simulink model "Cockpit"  (R2012b)
settings: Solver=ode45  StartTime=0.0  StopTime=10.0  RelTol=1e-3
undefined symbols (not defined in the file or in its folder): sigbuilder_block
libraries: vrlib x1
settings Model: Creator=David  LastModifiedBy=David

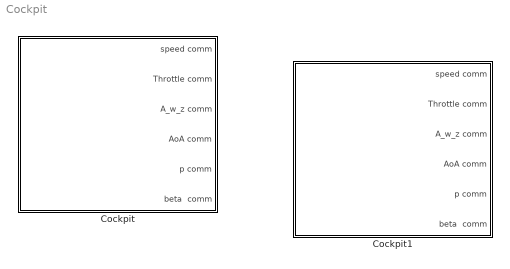
== system Cockpit ==
  Cockpit : Subsystem
      mask Display:
      | image(imread('Cockpit2.jpg'))
      | 
      | 
      | port_label('output', 1, 'Speed comm')
      | port_label('output', 2, 'Throttle comm')
      | port_label('output', 3, 'A_w_z comm')
      | port_label('output', 4, 'AoA comm')
      | port_label('output', 5, 'p comm')
      | port_label('output', 6, 'beta comm')
  Cockpit1 : Subsystem
      mask Display:
      | image(imread('Cockpit2.jpg'))
      | 
      | 
      | port_label('output', 1, 'Speed comm')
      | port_label('output', 2, 'Throttle comm')
      | port_label('output', 3, 'A_w_z comm')
      | port_label('output', 4, 'AoA comm')
      | port_label('output', 5, 'p comm')
      | port_label('output', 6, 'beta comm')

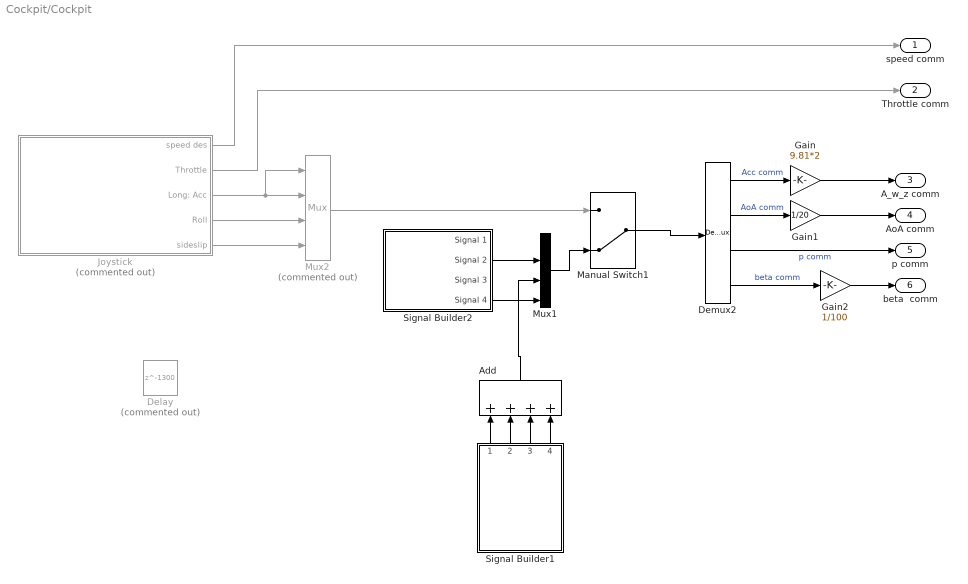
== system Cockpit/Cockpit ==
  Add : Sum  Inputs=++++
  Delay : Delay  Commented=on  DelayLength=1300
  Demux2 : Demux
  Gain : Gain  Gain=9.81*2
  Gain1 : Gain  Gain=1/20
  Gain2 : Gain  Gain=1/100
  Joystick : Subsystem  Commented=on
  Manual Switch1 : ManualSwitch  CurrentSetting=0
  Mux1 : Mux
  Mux2 : Mux  Commented=on
  Signal Builder1 : Subsystem  Tag=STV Subsys  LoadFcn=sigbuilder_block('load');  StartFcn=sigbuilder_block('start');  StopFcn=sigbuilder_block('stop');  ClipboardFcn=sigbuilder_block('clipboard');  mask(Sigbuilder block){}
      mask help: Simulink:masks:SigbuilderBlock_MD
      mask init:
      | if ~strcmp(get_param(bdroot(gcbh),'SimulationStatus'),'stopped') tuvar = sigbuilder_block('maskInit'); end
      settings: CopyFcn=sigbuilder_block('copy');  DeleteFcn=sigbuilder_block('delete');  ModelCloseFcn=sigbuilder_block('modelClose');  PreSaveFcn=sigbuilder_block('preSave');  PauseFcn=sigbuilder_block('pause');  ContinueFcn=sigbuilder_block('continue');  NameChangeFcn=sigbuilder_block('namechange');  OpenFcn=sigbuilder_block('open',[0 30 1024.5 489 ]);  CloseFcn=sigbuilder_block('close');
      mask Display: plot(0, 0, 100, 100,[2, 2, 32, 32, 2], [68, 8, 8, 68, 68],[32, 2], [38, 38], [32, 19, 2],[53, 60, 44], [32, 17, 17, 2],[16, 16, 31, 31]);txt = getActiveGroup(gcbh);text(2, 100, txt,'verticalAlignment', 'top');
  Signal Builder2 : Subsystem  Tag=STV Subsys  LoadFcn=sigbuilder_block('load');  StartFcn=sigbuilder_block('start');  StopFcn=sigbuilder_block('stop');  ClipboardFcn=sigbuilder_block('clipboard');  mask(Sigbuilder block){}
      mask help: Simulink:masks:SigbuilderBlock_MD
      mask init:
      | if ~strcmp(get_param(bdroot(gcbh),'SimulationStatus'),'stopped') tuvar = sigbuilder_block('maskInit'); end
      settings: CopyFcn=sigbuilder_block('copy');  DeleteFcn=sigbuilder_block('delete');  ModelCloseFcn=sigbuilder_block('modelClose');  PreSaveFcn=sigbuilder_block('preSave');  PauseFcn=sigbuilder_block('pause');  ContinueFcn=sigbuilder_block('continue');  NameChangeFcn=sigbuilder_block('namechange');  OpenFcn=sigbuilder_block('open',[6 28.5 1012.5 484.5 ]);  CloseFcn=sigbuilder_block('close');
      mask Display: plot(0, 0, 100, 100,[2, 2, 32, 32, 2], [68, 8, 8, 68, 68],[32, 2], [38, 38], [32, 19, 2],[53, 60, 44], [32, 17, 17, 2],[16, 16, 31, 31]);txt = getActiveGroup(gcbh);text(2, 100, txt,'verticalAlignment', 'top');
  speed comm : Outport
  Throttle comm : Outport  Port=2
  A_w_z comm : Outport  Port=3
  AoA comm : Outport  Port=4
  p comm : Outport  Port=5
  beta  comm : Outport  Port=6
  wires:
  Demux2/2 -> Gain1/1  "AoA comm"
  Gain/1 -> A_w_z comm/1
  Mux1/1 -> Manual Switch1/2
  Manual Switch1/1 -> Demux2/1
  Demux2/1 -> Gain/1  "Acc comm"
  Demux2/3 -> p comm/1  "p comm"
  Demux2/4 -> Gain2/1  "beta comm"
  Joystick/5(sideslip) -> Mux2/4
  Joystick/4(Roll) -> Mux2/3
  Joystick/2(Throttle) -> Throttle comm/1
  Mux2/1 -> Manual Switch1/1
  Joystick/3(Long: Acc) -> Mux2/1, Mux2/2
  Gain1/1 -> AoA comm/1
  Signal Builder1/1(Signal 1) -> Add/1
  Signal Builder1/2(Signal 5) -> Add/2
  Signal Builder1/4(Signal 7) -> Add/4
  Signal Builder1/3(Signal 6) -> Add/3
  Gain2/1 -> beta  comm/1
  Signal Builder2/2(Signal 2) -> Mux1/2
  Signal Builder2/4(Signal 4) -> Mux1/4
  Joystick/1(speed des) -> speed comm/1
  Add/1 -> Mux1/3

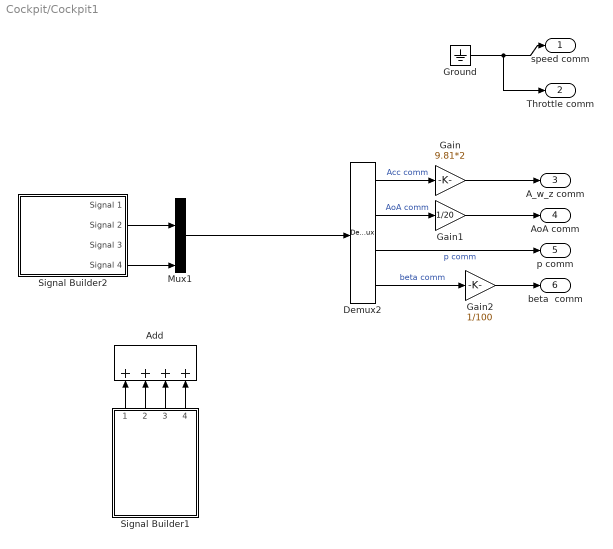
== system Cockpit/Cockpit1 ==
  Add : Sum  Inputs=++++
  Demux2 : Demux
  Gain : Gain  Gain=9.81*2
  Gain1 : Gain  Gain=1/20
  Gain2 : Gain  Gain=1/100
  Ground : Ground
  Mux1 : Mux
  Signal Builder1 : Subsystem  Tag=STV Subsys  LoadFcn=sigbuilder_block('load');  StartFcn=sigbuilder_block('start');  StopFcn=sigbuilder_block('stop');  ClipboardFcn=sigbuilder_block('clipboard');  mask(Sigbuilder block){}
      mask help: Simulink:masks:SigbuilderBlock_MD
      mask init:
      | if ~strcmp(get_param(bdroot(gcbh),'SimulationStatus'),'stopped') tuvar = sigbuilder_block('maskInit'); end
      settings: CopyFcn=sigbuilder_block('copy');  DeleteFcn=sigbuilder_block('delete');  ModelCloseFcn=sigbuilder_block('modelClose');  PreSaveFcn=sigbuilder_block('preSave');  PauseFcn=sigbuilder_block('pause');  ContinueFcn=sigbuilder_block('continue');  NameChangeFcn=sigbuilder_block('namechange');  OpenFcn=sigbuilder_block('open',[0 30 1024.5 489 ]);  CloseFcn=sigbuilder_block('close');
      mask Display: plot(0, 0, 100, 100,[2, 2, 32, 32, 2], [68, 8, 8, 68, 68],[32, 2], [38, 38], [32, 19, 2],[53, 60, 44], [32, 17, 17, 2],[16, 16, 31, 31]);txt = getActiveGroup(gcbh);text(2, 100, txt,'verticalAlignment', 'top');
  Signal Builder2 : Subsystem  Tag=STV Subsys  LoadFcn=sigbuilder_block('load');  StartFcn=sigbuilder_block('start');  StopFcn=sigbuilder_block('stop');  ClipboardFcn=sigbuilder_block('clipboard');  mask(Sigbuilder block){}
      mask help: Simulink:masks:SigbuilderBlock_MD
      mask init:
      | if ~strcmp(get_param(bdroot(gcbh),'SimulationStatus'),'stopped') tuvar = sigbuilder_block('maskInit'); end
      settings: CopyFcn=sigbuilder_block('copy');  DeleteFcn=sigbuilder_block('delete');  ModelCloseFcn=sigbuilder_block('modelClose');  PreSaveFcn=sigbuilder_block('preSave');  PauseFcn=sigbuilder_block('pause');  ContinueFcn=sigbuilder_block('continue');  NameChangeFcn=sigbuilder_block('namechange');  OpenFcn=sigbuilder_block('open',[6 28.5 1012.5 484.5 ]);  CloseFcn=sigbuilder_block('close');
      mask Display: plot(0, 0, 100, 100,[2, 2, 32, 32, 2], [68, 8, 8, 68, 68],[32, 2], [38, 38], [32, 19, 2],[53, 60, 44], [32, 17, 17, 2],[16, 16, 31, 31]);txt = getActiveGroup(gcbh);text(2, 100, txt,'verticalAlignment', 'top');
  speed comm : Outport
  Throttle comm : Outport  Port=2
  A_w_z comm : Outport  Port=3
  AoA comm : Outport  Port=4
  p comm : Outport  Port=5
  beta  comm : Outport  Port=6
  wires:
  Demux2/2 -> Gain1/1  "AoA comm"
  Gain/1 -> A_w_z comm/1
  Mux1/1 -> Demux2/1
  Demux2/1 -> Gain/1  "Acc comm"
  Demux2/3 -> p comm/1  "p comm"
  Demux2/4 -> Gain2/1  "beta comm"
  Gain1/1 -> AoA comm/1
  Signal Builder1/1(Signal 1) -> Add/1
  Signal Builder1/2(Signal 5) -> Add/2
  Signal Builder1/4(Signal 7) -> Add/4
  Signal Builder1/3(Signal 6) -> Add/3
  Gain2/1 -> beta  comm/1
  Signal Builder2/2(Signal 2) -> Mux1/2
  Signal Builder2/4(Signal 4) -> Mux1/4
  ? -> Mux1/3
  Ground/1 -> Throttle comm/1, speed comm/1

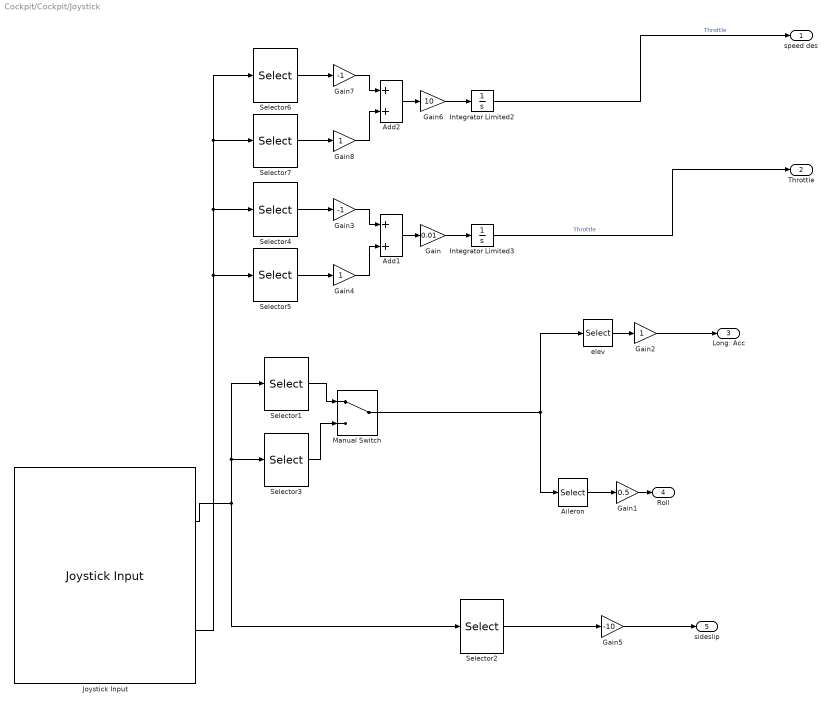
== system Cockpit/Cockpit/Joystick ==
  Add1 : Sum
  Add2 : Sum
  Aileron : Selector  InputPortWidth=2  IndexOptions=Index vector (dialog)  Indices=1  OutputSizes=1
  Gain : Gain  Gain=0.01  OutDataTypeStr=double
  Gain1 : Gain  Gain=0.5
  Gain2 : Gain
  Gain3 : Gain  Gain=-1
  Gain4 : Gain
  Gain5 : Gain  Gain=-10
  Gain6 : Gain  Gain=10  OutDataTypeStr=double
  Gain7 : Gain  Gain=-1
  Gain8 : Gain
  Integrator Limited2 : Integrator  LimitOutput=on  UpperSaturationLimit=400  LowerSaturationLimit=-400
  Integrator Limited3 : Integrator  LimitOutput=on  UpperSaturationLimit=1  LowerSaturationLimit=-1
  Joystick Input : vrlib/Joystick Input  joyid=1  adjustports=on  forcefeed=off
  Manual Switch : ManualSwitch
  Selector1 : Selector  InputPortWidth=5  IndexOptions=Index vector (dialog)  Indices=1:2  OutputSizes=1
  Selector2 : Selector  InputPortWidth=5  IndexOptions=Index vector (dialog)  Indices=3  OutputSizes=1
  Selector3 : Selector  InputPortWidth=5  IndexOptions=Index vector (dialog)  Indices=4:5  OutputSizes=1
  Selector4 : Selector  InputPortWidth=10  IndexOptions=Index vector (dialog)  Indices=1  OutputSizes=1
  Selector5 : Selector  InputPortWidth=10  IndexOptions=Index vector (dialog)  Indices=4  OutputSizes=1
  Selector6 : Selector  InputPortWidth=10  IndexOptions=Index vector (dialog)  Indices=1  OutputSizes=1
  Selector7 : Selector  InputPortWidth=10  IndexOptions=Index vector (dialog)  Indices=4  OutputSizes=1
  elev : Selector  InputPortWidth=2  IndexOptions=Index vector (dialog)  Indices=2  OutputSizes=1
  speed des : Outport
  Throttle : Outport  Port=2
  Long: Acc : Outport  Port=3
  Roll : Outport  Port=4
  sideslip : Outport  Port=5
  wires:
  Integrator Limited3/1 -> Throttle/1  "Throttle"
  Aileron/1 -> Gain1/1
  Manual Switch/1 -> Aileron/1, elev/1
  Joystick Input/1 -> Selector2/1, Selector3/1, Selector1/1
  Selector1/1 -> Manual Switch/1
  Selector3/1 -> Manual Switch/2
  Selector4/1 -> Gain3/1
  Selector5/1 -> Gain4/1
  Gain3/1 -> Add1/1
  Gain4/1 -> Add1/2
  Add1/1 -> Gain/1
  Gain/1 -> Integrator Limited3/1
  elev/1 -> Gain2/1
  Gain1/1 -> Roll/1
  Selector2/1 -> Gain5/1
  Gain2/1 -> Long: Acc/1
  Gain5/1 -> sideslip/1
  Integrator Limited2/1 -> speed des/1  "Throttle"
  Joystick Input/2 -> Selector5/1, Selector7/1, Selector6/1, Selector4/1
  Selector6/1 -> Gain7/1
  Selector7/1 -> Gain8/1
  Gain7/1 -> Add2/1
  Gain8/1 -> Add2/2
  Add2/1 -> Gain6/1
  Gain6/1 -> Integrator Limited2/1

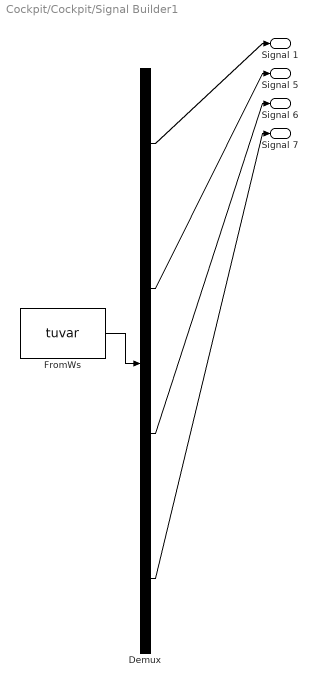
== system Cockpit/Cockpit/Signal Builder1 ==
  Demux : Demux  Tag=STV Demux
  FromWs : FromWorkspace  Tag=STV FromWs  VariableName=tuvar  SampleTime=0
      SigBuilderData=|
      | common.afterFinalStr = 'Extrapolate'
      | common.sampleTime = 0
      | dataSet.timeRange = [0 30]
      | dataSet.name = 'Group 1'
      | sbobj.Groups.Name = 'Group 1'
      | sbobj.Groups.Signals(1).Name = 'Signal 1'
      | sbobj.Groups.Signals(1).XData = [0 0.5 0.5 2.5 2.5 30]
      | sbobj.Groups.Signals(1).YData = [0 0 -1 -1 0 0]
      | sbobj.Groups.Signals(2).Name = 'Signal 5'
      | sbobj.Groups.Signals(2).XData = [0 4 4 6 6 30]
      | sbobj.Groups.Signals(2).YData = [0 0 1 1 0 0]
      | sbobj.Groups.Signals(3).Name = 'Signal 6'
      | sbobj.Groups.Signals(3).XData = [0 8 8 10 10 30]
      | sbobj.Groups.Signals(3).YData = [0 0 -0.5 -0.5 0 0]
      | sbobj.Groups.Signals(4).Name = 'Signal 7'
      | sbobj.Groups.Signals(4).XData = [0 12 12 14 14 30]
      | sbobj.Groups.Signals(4).YData = [0 0 0.5 0.5 0 0]
      | sbobj.Groups.TimeRange = [0 30]
  Signal 1 : Outport  Tag=STV Outport
  Signal 5 : Outport  Tag=STV Outport  Port=2
  Signal 6 : Outport  Tag=STV Outport  Port=3
  Signal 7 : Outport  Tag=STV Outport  Port=4
  wires:
  FromWs/1 -> Demux/1
  Demux/1 -> Signal 1/1
  Demux/2 -> Signal 5/1
  Demux/3 -> Signal 6/1
  Demux/4 -> Signal 7/1

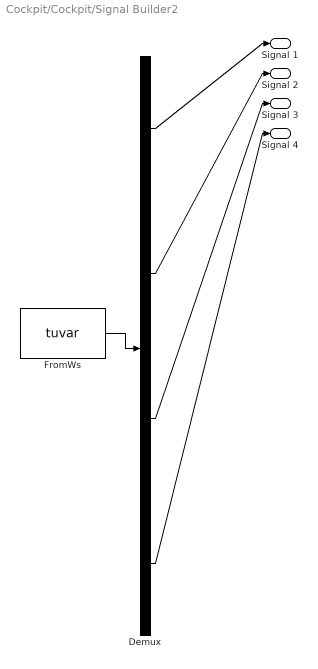
== system Cockpit/Cockpit/Signal Builder2 ==
  Demux : Demux  Tag=STV Demux
  FromWs : FromWorkspace  Tag=STV FromWs  VariableName=tuvar  SampleTime=0
      SigBuilderData=|
      | common.afterFinalStr = 'Extrapolate'
      | common.sampleTime = 0
      | dataSet.timeRange = [0 10]
      | dataSet.name = 'Group 1'
      | sbobj.Groups.Name = 'Group 1'
      | sbobj.Groups.Signals(1).Name = 'Signal 1'
      | sbobj.Groups.Signals(1).XData = [0 0.15 0.15 2.99 2.99 10]
      | sbobj.Groups.Signals(1).YData = [0 0 -1.07 -1.06 0.64 0.7]
      | sbobj.Groups.Signals(2).Name = 'Signal 2'
      | sbobj.Groups.Signals(2).XData = [0 10]
      | sbobj.Groups.Signals(2).YData = [0 0]
      | sbobj.Groups.Signals(3).Name = 'Signal 3'
      | sbobj.Groups.Signals(3).XData = [0 10]
      | sbobj.Groups.Signals(3).YData = [0 0]
      | sbobj.Groups.Signals(4).Name = 'Signal 4'
      | sbobj.Groups.Signals(4).XData = [0 10]
      | sbobj.Groups.Signals(4).YData = [0 0]
  Signal 1 : Outport  Tag=STV Outport
  Signal 2 : Outport  Tag=STV Outport  Port=2
  Signal 3 : Outport  Tag=STV Outport  Port=3
  Signal 4 : Outport  Tag=STV Outport  Port=4
  wires:
  FromWs/1 -> Demux/1
  Demux/1 -> Signal 1/1
  Demux/2 -> Signal 2/1
  Demux/3 -> Signal 3/1
  Demux/4 -> Signal 4/1

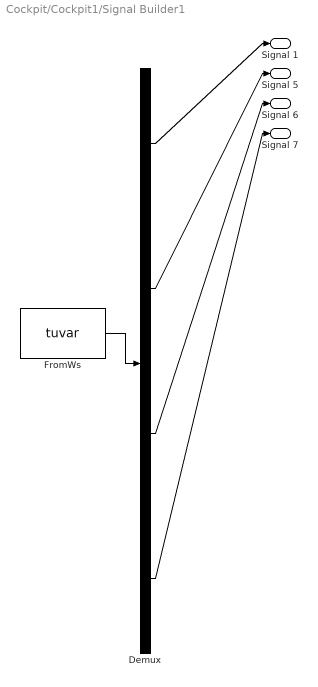
== system Cockpit/Cockpit1/Signal Builder1 ==
  Demux : Demux  Tag=STV Demux
  FromWs : FromWorkspace  Tag=STV FromWs  VariableName=tuvar  SampleTime=0
      SigBuilderData=|
      | common.afterFinalStr = 'Extrapolate'
      | common.sampleTime = 0
      | dataSet.timeRange = [0 30]
      | dataSet.name = 'Group 1'
      | sbobj.Groups.Name = 'Group 1'
      | sbobj.Groups.Signals(1).Name = 'Signal 1'
      | sbobj.Groups.Signals(1).XData = [0 0.5 0.5 2.5 2.5 30]
      | sbobj.Groups.Signals(1).YData = [0 0 -1 -1 0 0]
      | sbobj.Groups.Signals(2).Name = 'Signal 5'
      | sbobj.Groups.Signals(2).XData = [0 4 4 6 6 30]
      | sbobj.Groups.Signals(2).YData = [0 0 1 1 0 0]
      | sbobj.Groups.Signals(3).Name = 'Signal 6'
      | sbobj.Groups.Signals(3).XData = [0 8 8 10 10 30]
      | sbobj.Groups.Signals(3).YData = [0 0 -0.5 -0.5 0 0]
      | sbobj.Groups.Signals(4).Name = 'Signal 7'
      | sbobj.Groups.Signals(4).XData = [0 12 12 14 14 30]
      | sbobj.Groups.Signals(4).YData = [0 0 0.5 0.5 0 0]
      | sbobj.Groups.TimeRange = [0 30]
  Signal 1 : Outport  Tag=STV Outport
  Signal 5 : Outport  Tag=STV Outport  Port=2
  Signal 6 : Outport  Tag=STV Outport  Port=3
  Signal 7 : Outport  Tag=STV Outport  Port=4
  wires:
  FromWs/1 -> Demux/1
  Demux/1 -> Signal 1/1
  Demux/2 -> Signal 5/1
  Demux/3 -> Signal 6/1
  Demux/4 -> Signal 7/1

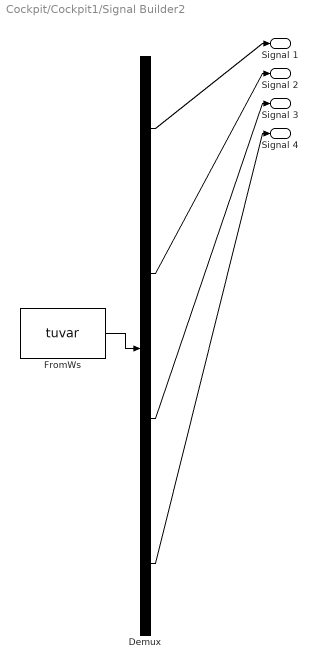
== system Cockpit/Cockpit1/Signal Builder2 ==
  Demux : Demux  Tag=STV Demux
  FromWs : FromWorkspace  Tag=STV FromWs  VariableName=tuvar  SampleTime=0
      SigBuilderData=|
      | common.afterFinalStr = 'Extrapolate'
      | common.sampleTime = 0
      | dataSet.timeRange = [0 10]
      | dataSet.name = 'Group 1'
      | sbobj.Groups.Name = 'Group 1'
      | sbobj.Groups.Signals(1).Name = 'Signal 1'
      | sbobj.Groups.Signals(1).XData = [0 0.15 0.15 2.99 2.99 10]
      | sbobj.Groups.Signals(1).YData = [0 0 -1.07 -1.06 0.64 0.7]
      | sbobj.Groups.Signals(2).Name = 'Signal 2'
      | sbobj.Groups.Signals(2).XData = [0 10]
      | sbobj.Groups.Signals(2).YData = [0 0]
      | sbobj.Groups.Signals(3).Name = 'Signal 3'
      | sbobj.Groups.Signals(3).XData = [0 10]
      | sbobj.Groups.Signals(3).YData = [0 0]
      | sbobj.Groups.Signals(4).Name = 'Signal 4'
      | sbobj.Groups.Signals(4).XData = [0 10]
      | sbobj.Groups.Signals(4).YData = [0 0]
  Signal 1 : Outport  Tag=STV Outport
  Signal 2 : Outport  Tag=STV Outport  Port=2
  Signal 3 : Outport  Tag=STV Outport  Port=3
  Signal 4 : Outport  Tag=STV Outport  Port=4
  wires:
  FromWs/1 -> Demux/1
  Demux/1 -> Signal 1/1
  Demux/2 -> Signal 2/1
  Demux/3 -> Signal 3/1
  Demux/4 -> Signal 4/1
